simulink model "LQR_SImulink_Ass_3"  (R2024b)
settings: Solver=VariableStepAuto  StartTime=0.0  StopTime=tf  RelTol=1e-3
values from neighbouring files (symbols this model uses):
  IC = [0;0; 0; 0]    [Main_Param_estimation.m]    (also in main.m)
  Wamp = 0    [Main_Param_estimation.m]    (also in main.m = 2)
settings Model: Creator=anton  LastModifiedBy=anton

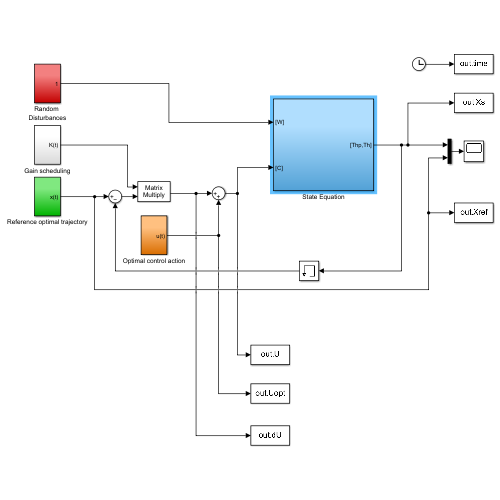
[thumbnail: Simulink's stored preview of the top-level diagram]
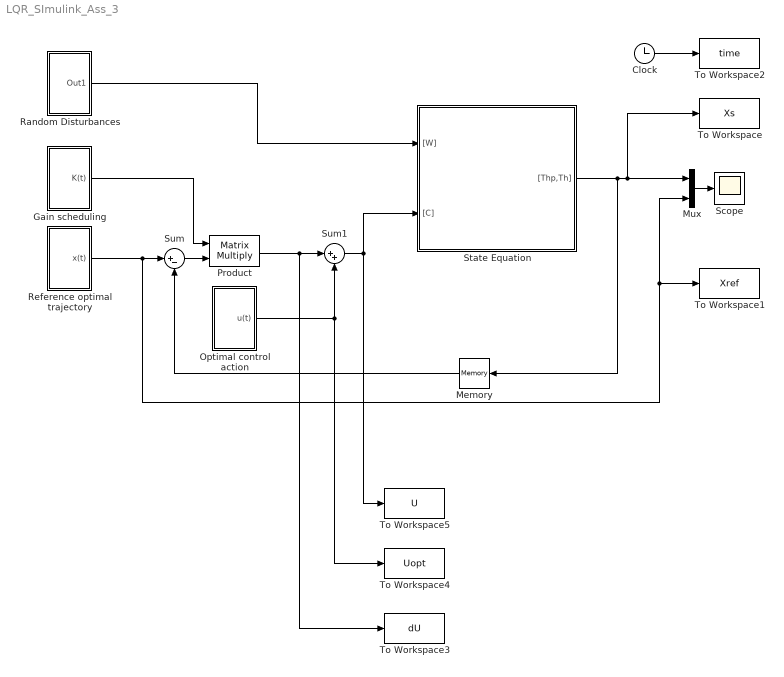
== system LQR_SImulink_Ass_3 ==
  Clock : Clock
  Gain scheduling : Subsystem
  Memory : Memory
  Mux : Mux  Inputs=2
  Optimal control action : Subsystem
  Product : Product  Multiplication=Matrix(*)
  Random Disturbances : Subsystem
  Reference optimal trajectory : Subsystem
  Scope : Scope
  State Equation : Subsystem
  Sum : Sum  Inputs=|+-
  Sum1 : Sum  Inputs=|++
  To Workspace : ToWorkspace  VariableName=Xs  SaveFormat=Timeseries  SampleTime=-1
  To Workspace1 : ToWorkspace  VariableName=Xref  SaveFormat=Timeseries  SampleTime=-1
  To Workspace2 : ToWorkspace  VariableName=time  SaveFormat=Timeseries  SampleTime=-1
  To Workspace3 : ToWorkspace  VariableName=dU  SaveFormat=Timeseries  SampleTime=-1
  To Workspace4 : ToWorkspace  VariableName=Uopt  SaveFormat=Timeseries  SampleTime=-1
  To Workspace5 : ToWorkspace  VariableName=U  SaveFormat=Timeseries  SampleTime=-1
  wires:
  Memory/1 -> Sum/2
  Reference optimal trajectory/1(x(t)) -> To Workspace1/1, Mux/2, Sum/1
  Optimal control action/1(u(t)) -> To Workspace4/1, Sum1/2
  Clock/1 -> To Workspace2/1
  Sum/1 -> Product/2
  Sum1/1 -> To Workspace5/1, State Equation/2("[C]")
  Gain scheduling/1(K(t)) -> Product/1
  State Equation/1("[Thp,Th]") -> To Workspace/1, Mux/1, Memory/1
  Mux/1 -> Scope/1
  Random Disturbances/1(Out1) -> State Equation/1("[W]")
  Product/1 -> Sum1/1, To Workspace3/1

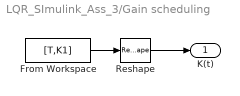
== system LQR_SImulink_Ass_3/Gain scheduling ==
  From Workspace : FromWorkspace  VariableName=[T,K1]
  Reshape : Reshape  OutputDimensionality=Row vector (2-D)
  K(t) : Outport
  wires:
  From Workspace/1 -> Reshape/1
  Reshape/1 -> K(t)/1

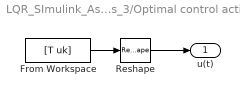
== system LQR_SImulink_Ass_3/Optimal control action ==
  From Workspace : FromWorkspace  VariableName=[T uk]
  Reshape : Reshape  OutputDimensionality=Column vector (2-D)
  u(t) : Outport
  wires:
  From Workspace/1 -> Reshape/1
  Reshape/1 -> u(t)/1

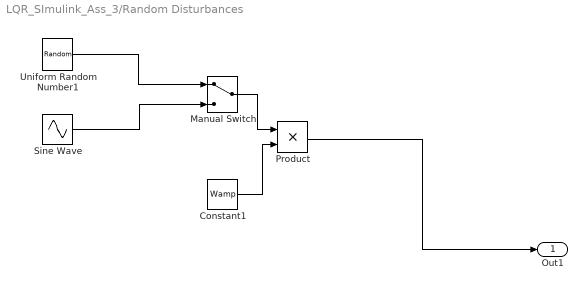
== system LQR_SImulink_Ass_3/Random Disturbances ==
  Constant1 : Constant  Value=Wamp
  Manual Switch : ManualSwitch
  Product : Product
  Sine Wave : Sin  Frequency=2*pi*100  SampleTime=0
  Uniform Random Number1 : UniformRandomNumber  SampleTime=tf/1000
  Out1 : Outport
  wires:
  Product/1 -> Out1/1
  Constant1/1 -> Product/2
  Uniform Random Number1/1 -> Manual Switch/1
  Sine Wave/1 -> Manual Switch/2
  Manual Switch/1 -> Product/1

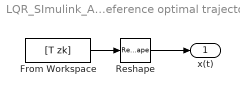
== system LQR_SImulink_Ass_3/Reference optimal trajectory ==
  From Workspace : FromWorkspace  VariableName=[T zk]
  Reshape : Reshape  OutputDimensionality=Column vector (2-D)
  x(t) : Outport
  wires:
  From Workspace/1 -> Reshape/1
  Reshape/1 -> x(t)/1

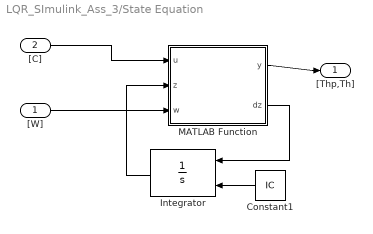
== system LQR_SImulink_Ass_3/State Equation ==
  "[W]" : Inport
  "[C]" : Inport  Port=2
  Constant1 : Constant  Value=IC
  Integrator : Integrator  InitialConditionSource=external
  MATLAB Function : MATLAB Function  TreatAsAtomicUnit=on
  "[Thp,Th]" : Outport
  wires:
  MATLAB Function/2(dz) -> Integrator/1
  Integrator/1 -> MATLAB Function/2(z)
  Constant1/1 -> Integrator/2
  MATLAB Function/1(y) -> "[Thp,Th]"/1
  "[C]"/1 -> MATLAB Function/1(u)
  "[W]"/1 -> MATLAB Function/3(w)

== matlab function LQR_SImulink_Ass_3/State Equation/MATLAB Function ==
  data: u input; z input; w input; y output; dz output
% function [y,dx]  = fcn(c,w,x)
% 
% m = 1;
% g = 9.81;
% L = 0.1;
% zeta = 0.02;
% w0 = sqrt(g/L);
% 
% dx = zeros(2,1);
% 
% u = c + w;
% 
% dx(1) = - 2*zeta*w0*x(1) - w0^2*sin(x(2)) + u/L^2/m;
% dx(2) = x(1);
% 
% y = [x(1);x(2)];


function [y, dz] = stateEq_new(u,z,w)

%% ========================================================================
% Funzione: stateEq_new
% ------------------------------------------------------------------------
% Descrizione:
%   Definisce le equazioni di stato del sistema dinamico non lineare.
%   Lo stato è composto da:
%       z = [x; y; θ; v]
%   dove:
%       x, y  → posizione
%       θ     → orientamento
%       v     → velocità
%   I controlli sono:
%       u1 → forza di trazione (accelerazione lungo la direzione θ)
%       u2 → controllo di rotazione (variazione dell'angolo θ)
%   Il modello include una resistenza aerodinamica proporzionale a v².
%
%   Equazioni:
%       ẋ = v*cos(θ)
%       ẏ = v*sin(θ)
%       θ̇ = u2
%       v̇ = (1/m)*(u1 - Cd*v²)
%
% Input:
%   t   → tempo corrente
%   z   → stato corrente [x; y; θ; v]
%   u   → controllo definito sulla griglia temporale Tu
%   Tu  → vettore temporale del controllo
%   m   → massa
%   Cd  → coefficiente di resistenza aerodinamica
%   w   → disturbo esterno
%
% Output:
%   dz  → derivata dello stato (vettore 4x1)
%% ========================================================================

    m   = 1;          % massa del corpo [kg]
    Cd  = 0.15;       % coefficiente di resistenza aerodinamica (attrito quadratico)

    dz = zeros(4,1);                     % inizializza derivata stato

    % Interpolazione dei controlli u1(t) e u2(t) al tempo corrente t
    u1 = u(1) + w;
    u2 = u(2) + w;

    % Equazioni dinamiche del sistema
    dz(1) = z(4)*cos(z(3));              % ẋ = v * cos(θ)
    dz(2) = z(4)*sin(z(3));              % ẏ = v * sin(θ)
    dz(3) = u2;                          % θ̇ = u2 (velocità angolare)
    dz(4) = 1/m*(u1 - Cd*z(4)^2);        % v̇ = (u1 - Cd*v²)/m

    y = [z(1); z(2); z(3); z(4)];

end
